simulink model "Simulacao"  (R2016b)
settings: Solver=VariableStepAuto  StartTime=0.0  StopTime=1000.0  RelTol=1e-3
InitFcn:
  | clc; clear;
  | main
values from neighbouring files (symbols this model uses):
  I = 900    [main.m]
  Tif = 70    [main.m]
  Tof = Tif + Tbarra    (= 85)    [main.m]
libraries: cstblocks x6
settings Model: Creator=tiago_lobao  LastModifiedBy=tiago_lobao

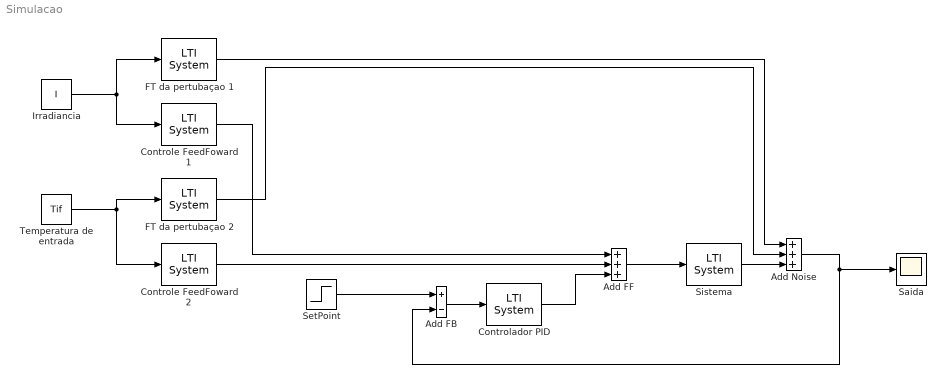
== system Simulacao ==
  "Add FB " : Sum  Inputs=+-
  Add FF : Sum  Inputs=+++
  "Add Noise " : Sum  Inputs=+++
  Controlador PID : cstblocks/LTI System  sys=C  IC=[]
  "Controle FeedFoward 1 " : cstblocks/LTI System  sys=Gff1  IC=[]
  Controle FeedFoward 2 : cstblocks/LTI System  sys=Gff2  IC=[]
  FT da pertubaçao 1 : cstblocks/LTI System  sys=P1  IC=[]
  FT da pertubaçao 2 : cstblocks/LTI System  sys=P2  IC=[]
  Irradiancia : Constant  Value=I
  Saida : Scope
  SetPoint : Step  After=Tof  SampleTime=0
  Sistema : cstblocks/LTI System  sys=G  IC=[]
  Temperatura de entrada : Constant  Value=Tif
  wires:
  SetPoint/1 -> "Add FB "/1
  Irradiancia/1 -> FT da pertubaçao 1/1, "Controle FeedFoward 1 "/1
  Temperatura de entrada/1 -> FT da pertubaçao 2/1, Controle FeedFoward 2/1
  Sistema/1 -> "Add Noise "/3
  FT da pertubaçao 1/1 -> "Add Noise "/1
  FT da pertubaçao 2/1 -> "Add Noise "/2
  "Add Noise "/1 -> "Add FB "/2, Saida/1
  "Controle FeedFoward 1 "/1 -> Add FF/1
  Controle FeedFoward 2/1 -> Add FF/2
  "Add FB "/1 -> Controlador PID/1
  Add FF/1 -> Sistema/1
  Controlador PID/1 -> Add FF/3
